simulink model "thrust_vector_rocket3_thrust"  (R2024b)
settings: Solver=VariableStepAuto  StartTime=0.0  StopTime=20.0  RelTol=1e-3
values from neighbouring files (symbols this model uses):
  A = [0 1; 0 0]    [model1_simplified.m]    (also in model2_no_thrustl.m = [0, 1, 0, 0, 0, 0; model3_thrust.m = [0, 1,      0, 0,       0, 0; model4_system_and_stability.m = jacobian(f, x))
  Axt = Ac(3:6, 3:6)    [model3_thrust.m]
  Ay = Ac(1:2, 1:2)    [model3_thrust.m]
  B = [0; -T*L/J]    [model1_simplified.m]    (also in model2_no_thrustl.m = [0; model3_thrust.m = [0   0; model4_system_and_stability.m = jacobian(f, u))
  Bxt = Bc(3:6, 2)    [model3_thrust.m]
  By = Bc(1:2, 1)    [model3_thrust.m]
  C = [1 0]    [model1_simplified.m]    (also in model2_no_thrustl.m = [1 0 0 0 0 0; model3_thrust.m = [1 0 0 0 0 0; model4_system_and_stability.m = [1 0 0 0 0 0)
  Cxt = [ 1     0     0     0 ... (first row only)    [model3_thrust.m]
  Cy = [1 0]    [model3_thrust.m]
  D = 0    [model1_simplified.m]    (also in model2_no_thrustl.m = [0; 0; 0]; model3_thrust.m = [0 0; 0 0; 0 0]; model4_system_and_stability.m)
  Dxt = [0; 0]    [model3_thrust.m]
  Dy = [0]    [model3_thrust.m]
  g = 9.81    [rocketParameters.mat]
  M = 1.5    [rocketParameters.mat]
  sys = ss(A,B,C,D)    [model1_simplified.m]    (also in model2_no_thrustl.m; model3_thrust.m; model4_system_and_stability.m = ss(A, B, eye(6), zeros(6,2)))
  Ts = 0.05    [model2_no_thrustl.m]    (also in model3_thrust.m; optimal_control.m; rocketParameters.mat)
  x0 = [0; 0; 0; 0; 5*pi/180; 0]    [model2_no_thrustl.m]    (also in model3_thrust.m)
  xf = zeros(6,1)    [model2_no_thrustl.m]    (also in model3_thrust.m = [0; 0; 2; 0; 0; 0])
libraries: slpidlib x3, mpclib x1
settings Model: Creator=wolfl  LastModifiedBy=wolfl

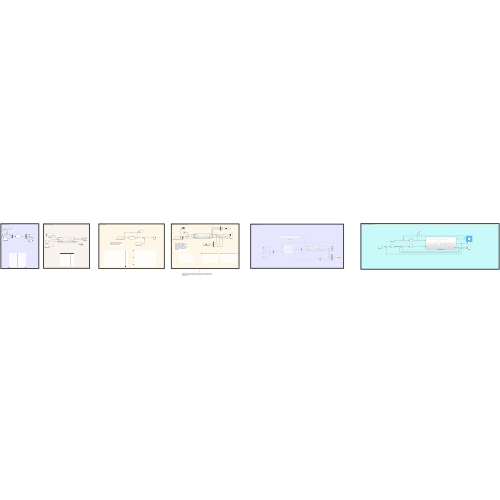
[thumbnail: Simulink's stored preview of the top-level diagram]
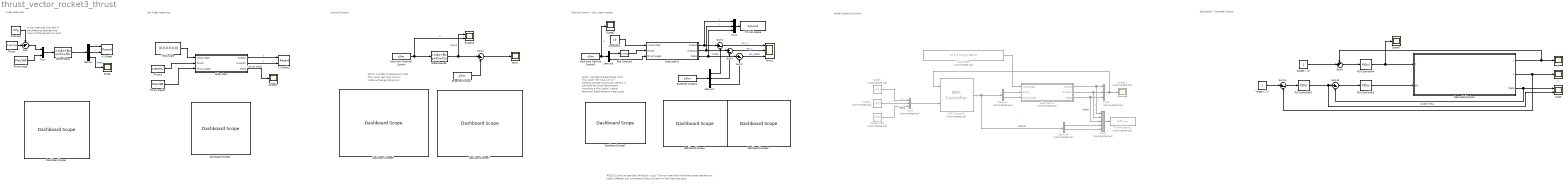
== system thrust_vector_rocket3_thrust ==
  note: Decoupled + Cascade Control
  note: RESULTS: We can see that the result is ugly! The non linearities make the system behave in a totally different way compared to the simulation in the linearized case
  note: In the linearized, the input is
      | the difference between the input
      | and the equilibrium point
  note: Non linear open-loop
  note: Linear open-loop
  note: NOTA: ricordati di selezionare "hold final value" nell'input, se no il sistema diverge malissimo!
  note: Optimal Control
  note: Optimal Control - Non Linear system
  note: NOTA: ricordati di selezionare "hold final value" nell'input, se no il sistema diverge malissimo!
      | NOTA2: Il controllo del thrust deve essere sommato a M*g, che è il valore attorno al quale abbiamo linearizzato
  note: Model Predictive Control
  Add Constant : Bias  Bias=M*g  SaturateOnIntegerOverflow=off
  Angle : Scope  NumInputPorts=2
  Constant : Constant  Value=M*g
  Constant1 : Constant  Value=x0
  Dashboard Scope{,1..5,7} (7 alike) : DashboardScope
  Decoupled System : Subsystem
  Demux : Demux  Outputs=3
  Demux1 : Demux  Commented=on  Outputs=2
  Demux2 : Demux  Outputs=3
  Demux3 : Demux  Outputs=2
  Demux5 : Demux  Commented=on  Outputs=2
  Error : Scope
  Error1 : Scope  NumInputPorts=3
  Expected Output : FromWorkspace  VariableName=ySim  OutputAfterFinalValue=Holding final value
  Expected Output1 : FromWorkspace  VariableName=ySim  OutputAfterFinalValue=Holding final value
  Initial State : Constant  Commented=on  Value=[0 0 0 0 5*pi/180 0]
  Input from Optimal Control : FromWorkspace  VariableName=uSim  SampleTime=Ts  OutputAfterFinalValue=Holding final value
  Input from Optimal Control1 : FromWorkspace  VariableName=uSim  SampleTime=Ts  OutputAfterFinalValue=Holding final value
  MPC Controller : mpclib/MPC Controller  Commented=on  SCDEnableBlockLinearizationSpecification=on  is_multiple=0  enable_value=0  return_u0=off  updateMPCinCallerWorkspace=on  md_inport=off  mv_inport=off  uref_inport=off  return_cost=off  return_mvseq=off  return_qpstatus=off  return_xseq=off  return_state=off  return_ovseq=off  state_inport=off  umin_inport=off  umax_inport=off  ymin_inport=off  ymax_inport=off  cc_inport=off  ywt_inport=off  uwt_inport=off  duwt_inport=off  rhoeps_inport=off  pm_inport=off  MaximumP=10  HorizonChoice=FixedHorizon  n_ts=0.05  n_p=10  n_mv=1  n_md=0  n_ud=0  n_mo=2  n_uo=0  BlockDataType=double  SampleTimeInherited=off  switch_inport=off
  Mux : Mux  Inputs=2
  Mux1 : Mux  Inputs=3
  Mux2 : Mux  Commented=on  Inputs=3
  Mux3 : Mux  Commented=on  Inputs=3
  Mux4 : Mux  Commented=on  Inputs=5
  PID Controller4 : slpidlib/PID Controller  Controller=PID  Form=Parallel  TimeDomain=Continuous-time  UseExternalTs=off  SampleTime=-1  IntegratorMethod=Forward Euler  FilterMethod=Forward Euler  ControllerParametersSource=internal  P=0.100224211410832  I=0.000848940546044858  UseKiTs=off  D=1.78175411585063  UseExternalDerivativeSource=off  N=135.692957961574  UseFilter=on  TunerSelectOption=Transfer Function Based (PID Tuner App)  InitialConditionSource=internal  InitialConditionForIntegrator=0  InitialConditionForFilter=0  DifferentiatorICPrevScaledInput=0  ExternalReset=none  TrackingMode=off  Kt=1  LimitOutput=off  SatLimitsSource=internal  UpperSaturationLimit=inf  LowerSaturationLimit=-inf  LinearizeAsGain=on  AntiWindupMode=none  Kb=1  LimitIntegrator=off  UpperIntegratorSaturationLimit=inf  LowerIntegratorSaturationLimit=-inf  POutMin=[]  POutMax=[]  IOutMin=[]  IOutMax=[]  DOutMin=[]  DOutMax=[]  NOutMin=[]  NOutMax=[]  SumOutMin=[]  SumOutMax=[]  SaturationOutMin=[]  SaturationOutMax=[]  PParamMin=[]  PParamMax=[]  IParamMin=[]  IParamMax=[]  DParamMin=[]  DParamMax=[]  NParamMin=[]  NParamMax=[]  KbParamMin=[]  KbParamMax=[]  KtParamMin=[]  KtParamMax=[]  KbOutMin=[]  KbOutMax=[]  KtOutMin=[]  KtOutMax=[]  IntegratorOutMin=[]  IntegratorOutMax=[]  FilterOutMin=[]  FilterOutMax=[]  SumI1OutMin=[]  SumI1OutMax=[]  SumI2OutMin=[]  SumI2OutMax=[]  SumI3OutMin=[]  SumI3OutMax=[]  SumI4OutMin=[]  SumI4OutMax=[]  SumDOutMin=[]  SumDOutMax=[]  DifferentiatorOutMin=[]  DifferentiatorOutMax=[]  FilterDiffOutCoefMin=[]  FilterDiffOutCoefMax=[]  ReciprocalOutMin=[]  ReciprocalOutMax=[]  SumDenOutMin=[]  SumDenOutMax=[]  SumNumOutMin=[]  SumNumOutMax=[]  DivideOutMin=[]  DivideOutMax=[]  UdiffTsProdOutMin=[]  UdiffTsProdOutMax=[]  NTsProdOutMin=[]  NTsProdOutMax=[]  UintegralTsProdOutMin=[]  UintegralTsProdOutMax=[]  UngainTsProdOutMin=[]  UngainTsProdOutMax=[]  ClampingZeroOutDataTypeStr=Inherit: Inherit via back propagation  ClampingZeroOutMin=[]  ClampingZeroOutMax=[]  FilterDenConstantOutDataTypeStr=Inherit: Inherit via back propagation  FilterDenConstantOutMin=[]  FilterDenConstantOutMax=[]  PCopyOutDataTypeStr=Inherit: Inherit via back propagation  PCopyOutMin=[]  PCopyOutMax=[]  NCopyOutDataTypeStr=Inherit: Inherit via back propagation  NCopyOutMin=[]  NCopyOutMax=[]  IntegratorContinuousStateAttributes=''  IntegratorStateMustResolveToSignalObject=off  IntegratorRTWStateStorageClass=Auto  FilterContinuousStateAttributes=''  FilterStateMustResolveToSignalObject=off  FilterRTWStateStorageClass=Auto  ParallelPVariant=InternalParameters  IdealPVariant=Disabled  IVariant=InternalParameters  DVariant=InternalParameters  IntegratorVariant=Continuous  SatVariant=Disabled  AWVariant=Passthrough  PCopyVariant=Disabled  TRVariant=Disabled  FdbkBlocksVariant=Forward  IdealPFdbkVariant=Disabled  SatFdbkVariant=Disabled  DerivativeFilterVariant=ContFilter  NVariant=InternalParameters  NCopyVariant=Disabled  FilterICVariant=InternalICsFilter  IntegratorICVariant=InternalICs  ExternalResetVariant=Disabled  TRSumVariant=Passthrough  SumFdbkVariant=Disabled  SumVariant=Sum_PID  TsampFilterVariant=InternalTs  TsampNgainVariant=Passthrough  TsampIntegralVariant=Disabled_SignalSpec  ExternalSaturationOutDataTypeStr=Inherit: Same as second input  DerivativeSourceVariant=ErrorSignal  PreIntVariant=InternalPreInt
  PID Controller5 : slpidlib/PID Controller  Controller=PID  Form=Parallel  TimeDomain=Continuous-time  UseExternalTs=off  SampleTime=-1  IntegratorMethod=Forward Euler  FilterMethod=Forward Euler  ControllerParametersSource=internal  P=-0.298828014391993  I=-0.102233083319818  UseKiTs=off  D=-0.200803156877234  UseExternalDerivativeSource=off  N=1142.8279760416  UseFilter=on  TunerSelectOption=Transfer Function Based (PID Tuner App)  InitialConditionSource=internal  InitialConditionForIntegrator=0  InitialConditionForFilter=0  DifferentiatorICPrevScaledInput=0  ExternalReset=none  TrackingMode=off  Kt=1  LimitOutput=off  SatLimitsSource=internal  UpperSaturationLimit=inf  LowerSaturationLimit=-inf  LinearizeAsGain=on  AntiWindupMode=none  Kb=1  LimitIntegrator=off  UpperIntegratorSaturationLimit=inf  LowerIntegratorSaturationLimit=-inf  POutMin=[]  POutMax=[]  IOutMin=[]  IOutMax=[]  DOutMin=[]  DOutMax=[]  NOutMin=[]  NOutMax=[]  SumOutMin=[]  SumOutMax=[]  SaturationOutMin=[]  SaturationOutMax=[]  PParamMin=[]  PParamMax=[]  IParamMin=[]  IParamMax=[]  DParamMin=[]  DParamMax=[]  NParamMin=[]  NParamMax=[]  KbParamMin=[]  KbParamMax=[]  KtParamMin=[]  KtParamMax=[]  KbOutMin=[]  KbOutMax=[]  KtOutMin=[]  KtOutMax=[]  IntegratorOutMin=[]  IntegratorOutMax=[]  FilterOutMin=[]  FilterOutMax=[]  SumI1OutMin=[]  SumI1OutMax=[]  SumI2OutMin=[]  SumI2OutMax=[]  SumI3OutMin=[]  SumI3OutMax=[]  SumI4OutMin=[]  SumI4OutMax=[]  SumDOutMin=[]  SumDOutMax=[]  DifferentiatorOutMin=[]  DifferentiatorOutMax=[]  FilterDiffOutCoefMin=[]  FilterDiffOutCoefMax=[]  ReciprocalOutMin=[]  ReciprocalOutMax=[]  SumDenOutMin=[]  SumDenOutMax=[]  SumNumOutMin=[]  SumNumOutMax=[]  DivideOutMin=[]  DivideOutMax=[]  UdiffTsProdOutMin=[]  UdiffTsProdOutMax=[]  NTsProdOutMin=[]  NTsProdOutMax=[]  UintegralTsProdOutMin=[]  UintegralTsProdOutMax=[]  UngainTsProdOutMin=[]  UngainTsProdOutMax=[]  ClampingZeroOutDataTypeStr=Inherit: Inherit via back propagation  ClampingZeroOutMin=[]  ClampingZeroOutMax=[]  FilterDenConstantOutDataTypeStr=Inherit: Inherit via back propagation  FilterDenConstantOutMin=[]  FilterDenConstantOutMax=[]  PCopyOutDataTypeStr=Inherit: Inherit via back propagation  PCopyOutMin=[]  PCopyOutMax=[]  NCopyOutDataTypeStr=Inherit: Inherit via back propagation  NCopyOutMin=[]  NCopyOutMax=[]  IntegratorContinuousStateAttributes=''  IntegratorStateMustResolveToSignalObject=off  IntegratorRTWStateStorageClass=Auto  FilterContinuousStateAttributes=''  FilterStateMustResolveToSignalObject=off  FilterRTWStateStorageClass=Auto  ParallelPVariant=InternalParameters  IdealPVariant=Disabled  IVariant=InternalParameters  DVariant=InternalParameters  IntegratorVariant=Continuous  SatVariant=Disabled  AWVariant=Passthrough  PCopyVariant=Disabled  TRVariant=Disabled  FdbkBlocksVariant=Forward  IdealPFdbkVariant=Disabled  SatFdbkVariant=Disabled  DerivativeFilterVariant=ContFilter  NVariant=InternalParameters  NCopyVariant=Disabled  FilterICVariant=InternalICsFilter  IntegratorICVariant=InternalICs  ExternalResetVariant=Disabled  TRSumVariant=Passthrough  SumFdbkVariant=Disabled  SumVariant=Sum_PID  TsampFilterVariant=InternalTs  TsampNgainVariant=Passthrough  TsampIntegralVariant=Disabled_SignalSpec  ExternalSaturationOutDataTypeStr=Inherit: Same as second input  DerivativeSourceVariant=ErrorSignal  PreIntVariant=InternalPreInt
  PID Controller6 : slpidlib/PID Controller  Controller=PID  Form=Parallel  TimeDomain=Continuous-time  UseExternalTs=off  SampleTime=-1  IntegratorMethod=Forward Euler  FilterMethod=Forward Euler  ControllerParametersSource=internal  P=-0.021217153772076  I=-0.00119437214783843  UseKiTs=off  D=-0.0895621821556866  UseExternalDerivativeSource=off  N=10.3067240404256  UseFilter=on  TunerSelectOption=Transfer Function Based (PID Tuner App)  InitialConditionSource=internal  InitialConditionForIntegrator=0  InitialConditionForFilter=0  DifferentiatorICPrevScaledInput=0  ExternalReset=none  TrackingMode=off  Kt=1  LimitOutput=off  SatLimitsSource=internal  UpperSaturationLimit=inf  LowerSaturationLimit=-inf  LinearizeAsGain=on  AntiWindupMode=none  Kb=1  LimitIntegrator=off  UpperIntegratorSaturationLimit=inf  LowerIntegratorSaturationLimit=-inf  POutMin=[]  POutMax=[]  IOutMin=[]  IOutMax=[]  DOutMin=[]  DOutMax=[]  NOutMin=[]  NOutMax=[]  SumOutMin=[]  SumOutMax=[]  SaturationOutMin=[]  SaturationOutMax=[]  PParamMin=[]  PParamMax=[]  IParamMin=[]  IParamMax=[]  DParamMin=[]  DParamMax=[]  NParamMin=[]  NParamMax=[]  KbParamMin=[]  KbParamMax=[]  KtParamMin=[]  KtParamMax=[]  KbOutMin=[]  KbOutMax=[]  KtOutMin=[]  KtOutMax=[]  IntegratorOutMin=[]  IntegratorOutMax=[]  FilterOutMin=[]  FilterOutMax=[]  SumI1OutMin=[]  SumI1OutMax=[]  SumI2OutMin=[]  SumI2OutMax=[]  SumI3OutMin=[]  SumI3OutMax=[]  SumI4OutMin=[]  SumI4OutMax=[]  SumDOutMin=[]  SumDOutMax=[]  DifferentiatorOutMin=[]  DifferentiatorOutMax=[]  FilterDiffOutCoefMin=[]  FilterDiffOutCoefMax=[]  ReciprocalOutMin=[]  ReciprocalOutMax=[]  SumDenOutMin=[]  SumDenOutMax=[]  SumNumOutMin=[]  SumNumOutMax=[]  DivideOutMin=[]  DivideOutMax=[]  UdiffTsProdOutMin=[]  UdiffTsProdOutMax=[]  NTsProdOutMin=[]  NTsProdOutMax=[]  UintegralTsProdOutMin=[]  UintegralTsProdOutMax=[]  UngainTsProdOutMin=[]  UngainTsProdOutMax=[]  ClampingZeroOutDataTypeStr=Inherit: Inherit via back propagation  ClampingZeroOutMin=[]  ClampingZeroOutMax=[]  FilterDenConstantOutDataTypeStr=Inherit: Inherit via back propagation  FilterDenConstantOutMin=[]  FilterDenConstantOutMax=[]  PCopyOutDataTypeStr=Inherit: Inherit via back propagation  PCopyOutMin=[]  PCopyOutMax=[]  NCopyOutDataTypeStr=Inherit: Inherit via back propagation  NCopyOutMin=[]  NCopyOutMax=[]  IntegratorContinuousStateAttributes=''  IntegratorStateMustResolveToSignalObject=off  IntegratorRTWStateStorageClass=Auto  FilterContinuousStateAttributes=''  FilterStateMustResolveToSignalObject=off  FilterRTWStateStorageClass=Auto  ParallelPVariant=InternalParameters  IdealPVariant=Disabled  IVariant=InternalParameters  DVariant=InternalParameters  IntegratorVariant=Continuous  SatVariant=Disabled  AWVariant=Passthrough  PCopyVariant=Disabled  TRVariant=Disabled  FdbkBlocksVariant=Forward  IdealPFdbkVariant=Disabled  SatFdbkVariant=Disabled  DerivativeFilterVariant=ContFilter  NVariant=InternalParameters  NCopyVariant=Disabled  FilterICVariant=InternalICsFilter  IntegratorICVariant=InternalICs  ExternalResetVariant=Disabled  TRSumVariant=Passthrough  SumFdbkVariant=Disabled  SumVariant=Sum_PID  TsampFilterVariant=InternalTs  TsampNgainVariant=Passthrough  TsampIntegralVariant=Disabled_SignalSpec  ExternalSaturationOutDataTypeStr=Inherit: Same as second input  DerivativeSourceVariant=ErrorSignal  PreIntVariant=InternalPreInt
  Scope{,1..2,7} (4 alike) : Scope
  Scope11 : Scope  NumInputPorts=2
  Scope12 : Scope  Commented=on
  State-Space : StateSpace  A=A  B=B  C=C  D=D  InitialCondition=[0, 0, 0, 0, 0, 0]
  State-Space3 : StateSpace  A=sys.a  B=sys.b  C=sys.c  D=sys.d  InitialCondition=x0
  Subsystem : Subsystem
  Subsystem1 : Subsystem
  Subsystem2 : Subsystem  Commented=on
  Sum : Sum  Inputs=-+|
  Sum{1..4,10..11} (6 alike) : Sum  Inputs=|+-
  Sum9 : Sum  Inputs=-+|
  Target theta : Constant  Commented=on  Value=xf(5)
  Target x : Constant  Commented=on  Value=xf(1)
  Target x (1) : Constant
  Target y : Constant  Commented=on  Value=xf(3)
  Target y (1) : Constant
  Thrust : Constant  Value=1.05*M*g
  Thrust angle : Constant  Value=0*pi/180
  Thrust angle1 : Constant  Value=0*pi/180
  Thrust1 : Constant  Value=1.05*M*g
  To Workspace : ToWorkspace  VariableName=simout1  SaveFormat=Timeseries  SampleTime=-1
  To Workspace1 : ToWorkspace  Commented=on  VariableName=MPCsim  SaveFormat=Timeseries  SampleTime=-1
  XY Graph : Record  FileSettingsInternal="{\"entries\":[{\"content\":{\"excelSettings\":{\"content\":{},\"type\":\"Streamout.ExcelSettings\"}},\"type\":\"Streamout.FileSettingStorage\",\"uuid\":\"\"}],\"packageUris\":[\"http:\\/\\/schema.mathworks.com\\/mf0\\/streamout_blocks\\/R2020a\"],\"version\":\"1.0\"}"  Layout=[1 1]  SignalsInternal="{\"entries\":[{\"content\":{\"signals\":[{\"content\":{\"blockPath\":[],\"dimensions\":[1],\"domain\":\"\",\"lineColor\":\"#edb120\",\"lineWidth\":2,\"plots\":[ 1 ],\"port\":1,\"sid\":[\"\"],\"signalID\":1,\"signalName\":\"x\"},\"type\":\"RecordBlkView.Signal\",\"uuid\":\"\"},{\"content\":{\"blockPath\":[],\"dimensions\":[1],\"domain\":\"\",\"lineColor\":\"#7e2f8e\",\"lineWidth\":2,\"plots\":[ 1 ],\"port\":2,\"sid\":[\"\"],\"signalID\":2,\"signalName\":\"y\"},\"type\":\"RecordBlkView.Signal\",\"uuid\":\"\"}]},\"type\":\"RecordBlkView.InputSignals\",\"uuid\":\"\"}],\"packageUris\":[\"http:\\/\\/schema.mathworks.com\\/mf0\\/streamout_blocks\\/R2020a\"],\"version\":\"1.0\"}"  VisualizationBindings="{\"xyplotplugin\":{\"info\":[{\"series\":[{\"bindingParametersList\":[{\"parameter\":\"X-Axis\",\"signalID\":1,\"signalName\":\"x\"},{\"parameter\":\"Y-Axis\",\"signalID\":2,\"signalName\":\"y\"}],\"seriesID\":0}],\"subplotID\":1}]}}"  CompatibilityTag=XY
  XY Graph1 : Record  FileSettingsInternal="{\"entries\":[{\"content\":{\"excelSettings\":{\"content\":{},\"type\":\"Streamout.ExcelSettings\"}},\"type\":\"Streamout.FileSettingStorage\",\"uuid\":\"\"}],\"packageUris\":[\"http:\\/\\/schema.mathworks.com\\/mf0\\/streamout_blocks\\/R2020a\"],\"version\":\"1.0\"}"  Layout=[1 1]  SignalsInternal="{\"entries\":[{\"content\":{\"signals\":[{\"content\":{\"blockPath\":[],\"dimensions\":[1],\"domain\":\"\",\"lineColor\":\"#77ac30\",\"lineWidth\":2,\"plots\":[ 1 ],\"port\":1,\"sid\":[\"\"],\"signalID\":1,\"signalName\":\"x\"},\"type\":\"RecordBlkView.Signal\",\"uuid\":\"\"},{\"content\":{\"blockPath\":[],\"dimensions\":[1],\"domain\":\"\",\"lineColor\":\"#4dbeee\",\"lineWidth\":2,\"plots\":[ 1 ],\"port\":2,\"sid\":[\"\"],\"signalID\":2,\"signalName\":\"y\"},\"type\":\"RecordBlkView.Signal\",\"uuid\":\"\"}]},\"type\":\"RecordBlkView.InputSignals\",\"uuid\":\"\"}],\"packageUris\":[\"http:\\/\\/schema.mathworks.com\\/mf0\\/streamout_blocks\\/R2020a\"],\"version\":\"1.0\"}"  VisualizationBindings="{\"xyplotplugin\":{\"info\":[{\"series\":[{\"bindingParametersList\":[{\"parameter\":\"X-Axis\",\"signalID\":1,\"signalName\":\"x\"},{\"parameter\":\"Y-Axis\",\"signalID\":2,\"signalName\":\"y\"}],\"seriesID\":0}],\"subplotID\":1}]}}"  CompatibilityTag=XY
  initial state : Constant  Value=[0,0,0,0,0,0]
  x : Scope
  y : Scope
  wires:
  Subsystem/2(Output1) -> XY Graph1/2  "y"
  Subsystem/1(Output) -> XY Graph1/1  "x"
  Demux/1 -> XY Graph/1  "x"
  initial state/1 -> Subsystem/1(initial state)
  Demux/2 -> XY Graph/2  "y"
  State-Space/1 -> Demux/1
  Demux/3 -> Scope/1  "theta"
  Thrust angle/1 -> Mux/2
  Subsystem/3(theta) -> Scope1/1  "rocket angle"
  Mux/1 -> State-Space/1
  Thrust/1 -> Sum/2
  Thrust1/1 -> Subsystem/2(thrust)
  Thrust angle1/1 -> Subsystem/3(thrust angle)
  Sum/1 -> Mux/1
  Constant/1 -> Sum/1
  Input from Optimal Control/1 -> State-Space3/1, Scope11/2  "u"
  State-Space3/1 -> Scope11/1, Sum4/1  "output"
  Sum4/1 -> Error/1
  Expected Output/1 -> Sum4/2
  Expected Output1/1 -> Demux2/1
  Sum1/1 -> Error1/1  "err_x"
  Demux3/2 -> Subsystem1/3(thrust angle)
  Add Constant/1 -> Subsystem1/2(thrust)
  Constant1/1 -> Subsystem1/1(initial state)
  Subsystem1/1(Output) -> Mux1/1, Sum1/1  "x"
  Subsystem1/2(Output1) -> Mux1/2, Sum2/1  "y"
  Subsystem1/3(theta) -> Mux1/3, Sum3/1  "theta"
  Demux2/1 -> Sum1/2
  Demux2/2 -> Sum2/2
  Demux2/3 -> Sum3/2
  Sum2/1 -> Error1/2  "err_y"
  Sum3/1 -> Error1/3  "err_theta"
  Mux1/1 -> To Workspace/1
  Input from Optimal Control1/1 -> Scope2/1, Demux3/1  "u"
  Demux3/1 -> Add Constant/1
  Initial State/1 -> Subsystem2/1(initial state)
  Target x/1 -> Mux2/1  "x"
  MPC Controller/1 -> Demux5/1, Demux1/1  "control"
  Target y/1 -> Mux2/2  "y"
  Target theta/1 -> Mux2/3  "theta"
  Mux2/1 -> MPC Controller/2
  Demux1/2 -> Subsystem2/3(thrust angle)
  Demux1/1 -> Subsystem2/2(thrust)
  Mux3/1 -> Scope12/1, MPC Controller/1
  Mux4/1 -> To Workspace1/1
  Subsystem2/2(Output1) -> Mux4/2, Mux3/2  "y"
  Subsystem2/1(Output) -> Mux4/1, Mux3/1  "x"
  Subsystem2/3(theta) -> Mux4/3, Mux3/3  "theta"
  Demux5/1 -> Mux4/4
  Demux5/2 -> Mux4/5
  Decoupled System/1(y) -> Sum9/1, y/1
  PID Controller4/1 -> Scope7/1, Decoupled System/1(T)
  Sum9/1 -> PID Controller4/1
  Target y (1)/1 -> Sum9/2
  Sum10/1 -> PID Controller5/1
  PID Controller5/1 -> Decoupled System/2(phi)
  Decoupled System/3(theta) -> Angle/1, Sum10/2
  Decoupled System/2(x) -> x/1, Sum11/2
  Target x (1)/1 -> Sum11/1
  Sum11/1 -> PID Controller6/1
  PID Controller6/1 -> Angle/2, Sum10/1  "target theta"

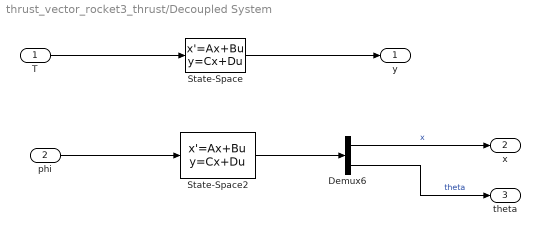
== system thrust_vector_rocket3_thrust/Decoupled System ==
  T : Inport
  phi : Inport  Port=2
  Demux6 : Demux  Outputs=2
  State-Space : StateSpace  A=Ay  B=By  C=Cy  D=Dy  InitialCondition=[0, 0]
  State-Space2 : StateSpace  A=Axt  B=Bxt  C=Cxt  D=Dxt  InitialCondition=[0 0 0 0]
  y : Outport
  x : Outport  Port=2
  theta : Outport  Port=3
  wires:
  State-Space/1 -> y/1
  T/1 -> State-Space/1
  phi/1 -> State-Space2/1
  Demux6/1 -> x/1  "x"
  State-Space2/1 -> Demux6/1
  Demux6/2 -> theta/1  "theta"

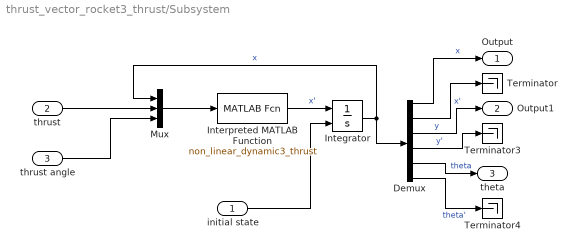
== system thrust_vector_rocket3_thrust/Subsystem ==
  initial state : Inport
  thrust : Inport  Port=2
  thrust angle : Inport  Port=3
  Demux : Demux  Outputs=6
  Integrator : Integrator  InitialConditionSource=external
  Interpreted MATLAB Function : MATLABFcn  MATLABFcn=non_linear_dynamic3_thrust
  Mux : Mux  Inputs=3
  Terminator : Terminator
  Terminator3 : Terminator
  Terminator4 : Terminator
  Output : Outport
  Output1 : Outport  Port=2
  theta : Outport  Port=3
  wires:
  thrust/1 -> Mux/2
  Interpreted MATLAB Function/1 -> Integrator/1  "x'"
  Mux/1 -> Interpreted MATLAB Function/1
  Demux/1 -> Output/1  "x"
  Demux/2 -> Terminator/1  "x'"
  Integrator/1 -> Mux/1, Demux/1  "x"
  initial state/1 -> Integrator/2
  Demux/3 -> Output1/1  "y"
  Demux/4 -> Terminator3/1  "y'"
  Demux/5 -> theta/1  "theta"
  Demux/6 -> Terminator4/1  "theta'"
  thrust angle/1 -> Mux/3

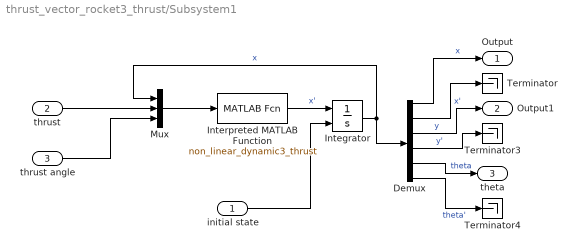
== system thrust_vector_rocket3_thrust/Subsystem1 ==
  initial state : Inport
  thrust : Inport  Port=2
  thrust angle : Inport  Port=3
  Demux : Demux  Outputs=6
  Integrator : Integrator  InitialConditionSource=external
  Interpreted MATLAB Function : MATLABFcn  MATLABFcn=non_linear_dynamic3_thrust
  Mux : Mux  Inputs=3
  Terminator : Terminator
  Terminator3 : Terminator
  Terminator4 : Terminator
  Output : Outport
  Output1 : Outport  Port=2
  theta : Outport  Port=3
  wires:
  thrust/1 -> Mux/2
  Interpreted MATLAB Function/1 -> Integrator/1  "x'"
  Mux/1 -> Interpreted MATLAB Function/1
  Demux/1 -> Output/1  "x"
  Demux/2 -> Terminator/1  "x'"
  Integrator/1 -> Mux/1, Demux/1  "x"
  initial state/1 -> Integrator/2
  Demux/3 -> Output1/1  "y"
  Demux/4 -> Terminator3/1  "y'"
  Demux/5 -> theta/1  "theta"
  Demux/6 -> Terminator4/1  "theta'"
  thrust angle/1 -> Mux/3

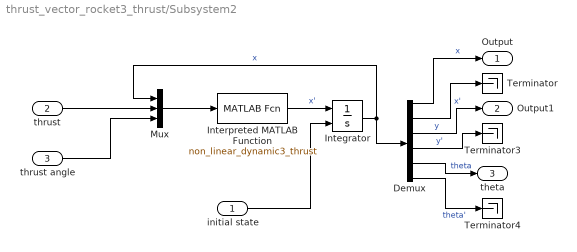
== system thrust_vector_rocket3_thrust/Subsystem2 ==
  initial state : Inport
  thrust : Inport  Port=2
  thrust angle : Inport  Port=3
  Demux : Demux  Outputs=6
  Integrator : Integrator  InitialConditionSource=external
  Interpreted MATLAB Function : MATLABFcn  MATLABFcn=non_linear_dynamic3_thrust
  Mux : Mux  Inputs=3
  Terminator : Terminator
  Terminator3 : Terminator
  Terminator4 : Terminator
  Output : Outport
  Output1 : Outport  Port=2
  theta : Outport  Port=3
  wires:
  thrust/1 -> Mux/2
  Interpreted MATLAB Function/1 -> Integrator/1  "x'"
  Mux/1 -> Interpreted MATLAB Function/1
  Demux/1 -> Output/1  "x"
  Demux/2 -> Terminator/1  "x'"
  Integrator/1 -> Mux/1, Demux/1  "x"
  initial state/1 -> Integrator/2
  Demux/3 -> Output1/1  "y"
  Demux/4 -> Terminator3/1  "y'"
  Demux/5 -> theta/1  "theta"
  Demux/6 -> Terminator4/1  "theta'"
  thrust angle/1 -> Mux/3
